simulink model "OswaldE_Project4_Sim"  (R2024b)
settings: Solver=VariableStepAuto  StartTime=0.0  StopTime=20  RelTol=1e-3
values from neighbouring files (symbols this model uses):
  K = place(plant.generalized.A, plant.generalized.B, p)    [OswaldE_Project4_Code.m]
  K5 = 0.5    [OswaldE_Project4_Code.m]
  step_size = 0.015 * i    [OswaldE_Project4_Code.m]
undefined symbols (not defined in the file or in its folder): trim
libraries: cstblocks x2
settings Model: Creator=ethan  LastModifiedBy=ethan

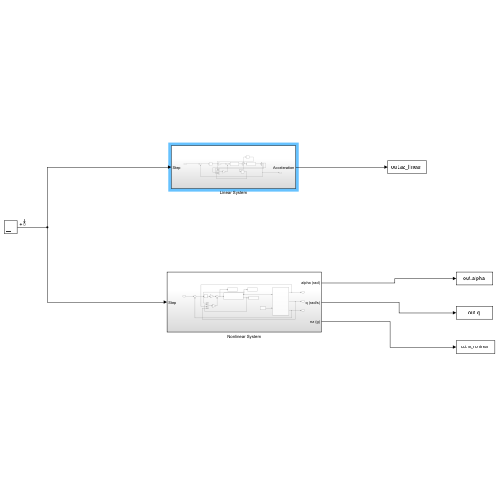
[thumbnail: Simulink's stored preview of the top-level diagram]
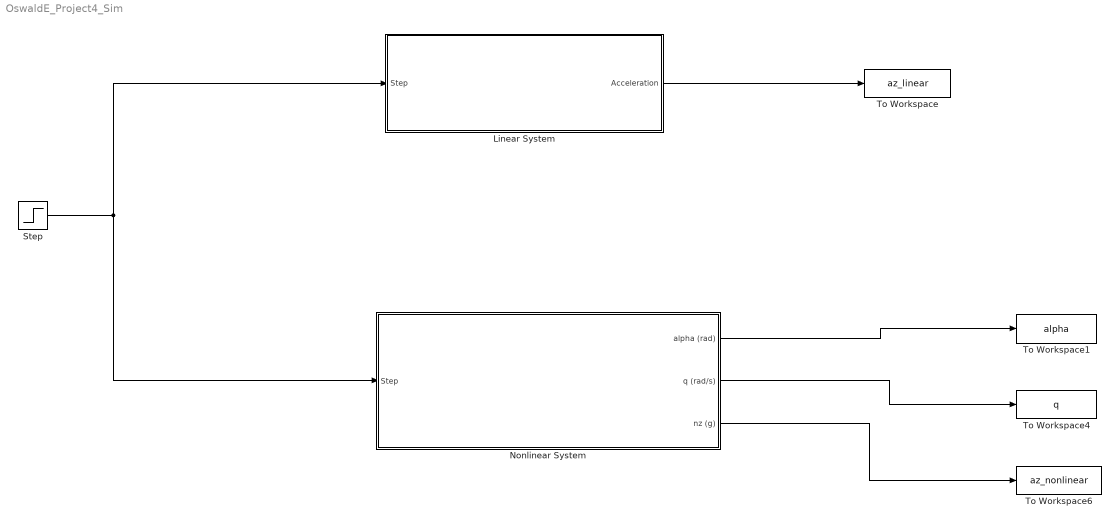
== system OswaldE_Project4_Sim ==
  Linear System : Subsystem
  Nonlinear System : Subsystem
  Step : Step  Time=0  After=step_size  SampleTime=0
  To Workspace : ToWorkspace  VariableName=az_linear  SaveFormat=Timeseries  SampleTime=-1
  To Workspace1 : ToWorkspace  VariableName=alpha  SampleTime=-1
  To Workspace4 : ToWorkspace  VariableName=q  SampleTime=-1
  To Workspace6 : ToWorkspace  VariableName=az_nonlinear  SaveFormat=Timeseries  SampleTime=-1
  wires:
  Step/1 -> Nonlinear System/1(Step), Linear System/1(Step)
  Linear System/1(Acceleration) -> To Workspace/1
  Nonlinear System/1(alpha (rad)) -> To Workspace1/1
  Nonlinear System/2(q (rad/s)) -> To Workspace4/1
  Nonlinear System/3(nz (g)) -> To Workspace6/1

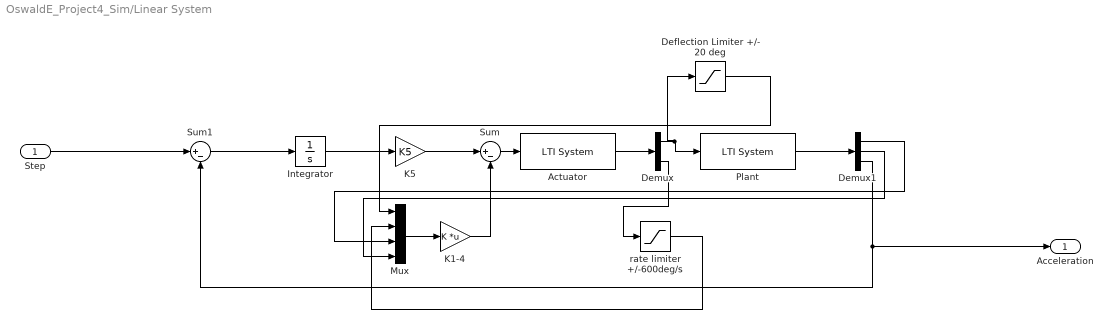
== system OswaldE_Project4_Sim/Linear System ==
  Step : Inport
  Actuator : cstblocks/LTI System  sys=actuator.ss  IC=[]  PadeOrder=0
  Deflection Limiter +/- 20 deg : Saturate  UpperLimit=20*pi/180  LowerLimit=-20*pi/180
  Demux : Demux  Outputs=2
  Demux1 : Demux  Outputs=3
  Integrator : Integrator
  K1-4 : Gain  Gain=K  Multiplication=Matrix(K*u)
  K5 : Gain  Gain=K5
  Mux : Mux
  Plant : cstblocks/LTI System  sys=plant.ss  IC=[]  PadeOrder=0
  Sum : Sum  Inputs=|+-
  Sum1 : Sum  Inputs=|+-
  rate limiter +/-600deg/s : Saturate  UpperLimit=600*pi/180  LowerLimit=-600*pi/180
  Acceleration : Outport
  wires:
  Sum/1 -> Actuator/1
  K1-4/1 -> Sum/2
  Sum1/1 -> Integrator/1
  Demux/2 -> rate limiter +/-600deg/s/1
  Demux/1 -> Deflection Limiter +/- 20 deg/1, Plant/1
  rate limiter +/-600deg/s/1 -> Mux/2
  Demux1/1 -> Mux/3
  Integrator/1 -> K5/1
  Plant/1 -> Demux1/1
  Deflection Limiter +/- 20 deg/1 -> Mux/1
  Demux1/3 -> Acceleration/1, Sum1/2
  Actuator/1 -> Demux/1
  K5/1 -> Sum/1
  Demux1/2 -> Mux/4
  Mux/1 -> K1-4/1
  Step/1 -> Sum1/1

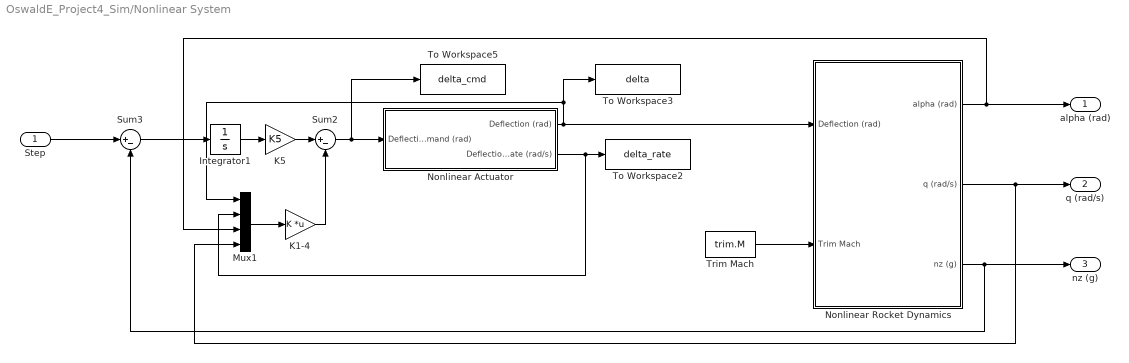
== system OswaldE_Project4_Sim/Nonlinear System ==
  Step : Inport
  Integrator1 : Integrator
  K1-4 : Gain  Gain=K  Multiplication=Matrix(K*u)
  K5 : Gain  Gain=K5
  Mux1 : Mux
  Nonlinear Actuator : Subsystem
  Nonlinear Rocket Dynamics : Subsystem
  Sum2 : Sum  Inputs=|+-
  Sum3 : Sum  Inputs=|+-
  To Workspace2 : ToWorkspace  VariableName=delta_rate  SampleTime=-1
  To Workspace3 : ToWorkspace  VariableName=delta  SampleTime=-1
  To Workspace5 : ToWorkspace  VariableName=delta_cmd  SampleTime=-1
  Trim Mach : Constant  Value=trim.M
  alpha (rad) : Outport
  q (rad/s) : Outport  Port=2
  nz (g) : Outport  Port=3
  wires:
  Nonlinear Actuator/2(Deflection Rate (rad/s)) -> Mux1/2, To Workspace2/1
  K1-4/1 -> Sum2/2
  Trim Mach/1 -> Nonlinear Rocket Dynamics/2(Trim Mach)
  Sum2/1 -> To Workspace5/1, Nonlinear Actuator/1(Deflection command (rad))
  Nonlinear Actuator/1(Deflection (rad)) -> Nonlinear Rocket Dynamics/1(Deflection (rad)), To Workspace3/1, Mux1/1
  Integrator1/1 -> K5/1
  Nonlinear Rocket Dynamics/3(nz (g)) -> nz (g)/1, Sum3/2
  Nonlinear Rocket Dynamics/2(q (rad/s)) -> q (rad/s)/1, Mux1/4
  Mux1/1 -> K1-4/1
  K5/1 -> Sum2/1
  Sum3/1 -> Integrator1/1
  Nonlinear Rocket Dynamics/1(alpha (rad)) -> alpha (rad)/1, Mux1/3
  Step/1 -> Sum3/1

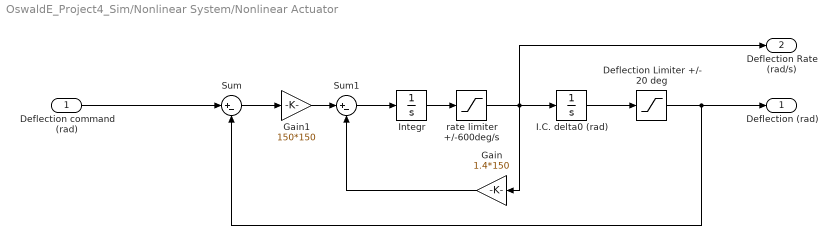
== system OswaldE_Project4_Sim/Nonlinear System/Nonlinear Actuator ==
  Deflection command (rad) : Inport
  Deflection Limiter +/- 20 deg : Saturate  UpperLimit=20*pi/180  LowerLimit=-20*pi/180
  Gain : Gain  Gain=1.4*150
  Gain1 : Gain  Gain=150*150
  I.C. delta0 (rad) : Integrator
  Integr : Integrator
  Sum : Sum  Inputs=|+-
  Sum1 : Sum  Inputs=|+-
  rate limiter +/-600deg/s : Saturate  UpperLimit=600*pi/180  LowerLimit=-600*pi/180
  Deflection (rad) : Outport
  Deflection Rate (rad/s) : Outport  Port=2
  wires:
  Integr/1 -> rate limiter +/-600deg/s/1
  Deflection command (rad)/1 -> Sum/1
  Sum1/1 -> Integr/1
  Gain/1 -> Sum1/2
  Gain1/1 -> Sum1/1
  rate limiter +/-600deg/s/1 -> I.C. delta0 (rad)/1, Deflection Rate (rad/s)/1, Gain/1
  Deflection Limiter +/- 20 deg/1 -> Deflection (rad)/1, Sum/2
  I.C. delta0 (rad)/1 -> Deflection Limiter +/- 20 deg/1
  Sum/1 -> Gain1/1

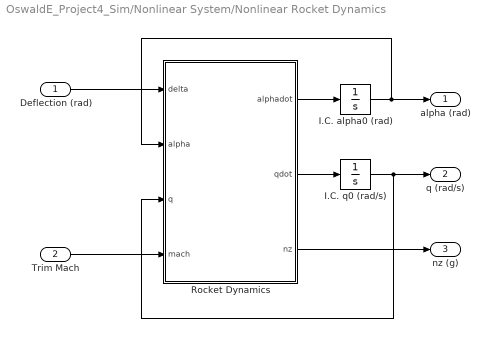
== system OswaldE_Project4_Sim/Nonlinear System/Nonlinear Rocket Dynamics ==
  Deflection (rad) : Inport
  Trim Mach : Inport  Port=2
  I.C. alpha0 (rad) : Integrator
  I.C. q0 (rad/s) : Integrator
  Rocket Dynamics : MATLAB Function  TreatAsAtomicUnit=on
  alpha (rad) : Outport
  q (rad/s) : Outport  Port=2
  nz (g) : Outport  Port=3
  wires:
  Rocket Dynamics/3(nz) -> nz (g)/1
  I.C. alpha0 (rad)/1 -> Rocket Dynamics/2(alpha), alpha (rad)/1
  I.C. q0 (rad/s)/1 -> q (rad/s)/1, Rocket Dynamics/3(q)
  Deflection (rad)/1 -> Rocket Dynamics/1(delta)
  Trim Mach/1 -> Rocket Dynamics/4(mach)
  Rocket Dynamics/1(alphadot) -> I.C. alpha0 (rad)/1
  Rocket Dynamics/2(qdot) -> I.C. q0 (rad/s)/1

== matlab function OswaldE_Project4_Sim/Nonlinear System/Nonlinear Rocket Dynamics/Rocket Dynamics ==
  data: delta input; alpha input; q input; alphadot output; qdot output; nz output; mach input
function [alphadot, qdot, nz] = rocket_dynamics(delta, alpha, q, mach)

% Unit conversion factors
d2r = pi/180;               % Degrees to radians
r2d = 1/d2r;                % Radians to degrees

% Aircraft Parameters
p_s = 973.3;         % Static pressure at 20000ft, lbs/ft^2
c_s = 1036.4;        % Speed of sound at 20000ft, ft/sec
S_ref = 0.44;        % Reference area, ft^2
d = 0.75;            % Diameter, ft
mass = 13.98;        % Mass, slugs
inertia_y = 182.5;   % Pitch moment of inertia, slug*ft^2
gravity = 32.2;      % Gravitational acceleration, ft/sec^2

% Aerodynamic coefficients for Cn and Cm: See project file for more
% details. The coefficients n1 and m1 depend on Mach number as:
%   n1 = n1a+n1b*Mach
%   m1 = m1a+m1b*Mach
n0= -0.034*r2d; 
n2= -9.4457e-3*r2d^2; 
n3 = 0.000103*r2d^3;
m0= -0.206*r2d; 
m2= -1.9546e-2*r2d^2;
m3 = 0.000215*r2d^3;

n1a = -2*0.1696*r2d;
n1b = 0.1696/3*r2d;

m1a =  -7*0.051*r2d;
m1b =  8/3*0.051*r2d;

% Dynamic pressure and airspeed
dynamic_pressure = 0.7*p_s*mach^2;

% Remaining aero coefficients at specified Mach number
n1 = n1a+n1b*mach;
m1 = m1a+m1b*mach;

% Aerodynamic Forces
force_coef = sign(alpha)*(n3*abs(alpha)^3 + n2*alpha^2 + ...
    n1*abs(alpha)) + n0*delta;
moment_coef = sign(alpha)*(m3*abs(alpha)^3 + m2*alpha^2 + ...
    m1*abs(alpha)) + m0*delta;
vertical_force = force_coef*dynamic_pressure*S_ref;
y_moment = moment_coef *dynamic_pressure*S_ref*d;

% compute alphadot and qdot vector
alphadot = cos(alpha)*vertical_force/(mass*mach*c_s) + q;
qdot = y_moment/inertia_y;
nz = d2r*vertical_force/(mass*gravity);
